simulink model "Lab3_2"  (R2016a)
settings: Solver=FixedStepDiscrete  StartTime=0.0  StopTime=10.0  RelTol=1e-3
settings Model: Creator=NoteBook  LastModifiedBy=NoteBook
settings OptimizationCC: DefaultParameterBehavior=Inlined  EnableMemcpy=off  OptimizeModelRefInitCode=on  LifeSpan=1
settings DebuggingCC: UnderspecifiedInitializationDetection=Classic  MergeDetectMultiDrivingBlocksExec=none
settings ModelReferenceCC: PropagateSignalLabelsOutOfModel=off
settings RTWCC: SystemTargetFile=ert.tlc  GenCodeOnly=on  TemplateMakefile=ert_default_tmf  GenerateReport=on  IncludeHyperlinkInReport=on  LaunchReport=on  GenerateTraceInfo=on  GenerateTraceReport=on  GenerateTraceReportSl=on  GenerateTraceReportSf=on  GenerateTraceReportEml=on
settings CodeAppCC: ForceParamTrailComments=on  IgnoreCustomStorageClasses=off  OperatorAnnotations=on  SimulinkDataObjDesc=on  SFDataObjDesc=on  MATLABFcnDesc=on  InsertBlockDesc=on  MATLABSourceComments=on
settings ERTTargetCC: GenerateSampleERTMain=on  InlinedParameterPlacement=NonHierarchical  ERTCustomFileTemplate=example_file_process.tlc

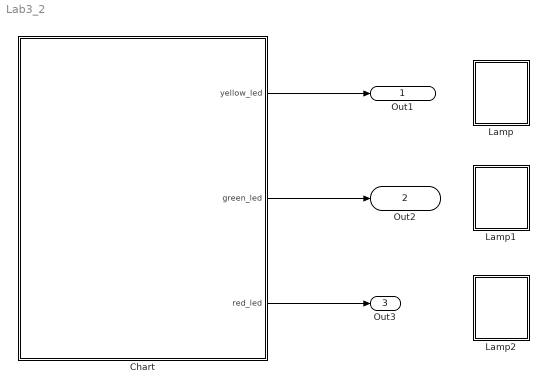
== system Lab3_2 ==
  Chart : Stateflow chart  TreatAsAtomicUnit=on
  Lamp : Subsystem  DialogController=hmiCreateDDGDialog  IsWebBlock=on  mask(MWDashboardBlock){webBlockId=2661d3e9-8543-4f99-aaf3-ccca5fb902ba, webBlockType=lamp, ShowInLibBrowser=on, ShowInitialText=on, HMISrcModelName=Lab3_2}
      mask prompts: webBlockType "WebBlock Type"; HMISrcModelName "Source Model"
      mask Help: helpview([docroot '/mapfiles/simulink.map'], 'hmi_lamp')
      mask Display:
      | if strcmp(get_param(bdroot(gcb),'BlockDiagramType'), 'library')
      |     image([(matlabroot) '/toolbox/simulink/hmi/icons/Lamp.png']);
      | end
  Lamp1 : Subsystem  DialogController=hmiCreateDDGDialog  IsWebBlock=on  mask(MWDashboardBlock){webBlockId=5fd369d1-2967-4dad-81f1-e6972ce0e81c, webBlockType=lamp, ShowInLibBrowser=on, ShowInitialText=on, HMISrcModelName=Lab3_2}
      mask prompts: webBlockType "WebBlock Type"; HMISrcModelName "Source Model"
      mask Help: helpview([docroot '/mapfiles/simulink.map'], 'hmi_lamp')
      mask Display:
      | if strcmp(get_param(bdroot(gcb),'BlockDiagramType'), 'library')
      |     image([(matlabroot) '/toolbox/simulink/hmi/icons/Lamp.png']);
      | end
  Lamp2 : Subsystem  DialogController=hmiCreateDDGDialog  IsWebBlock=on  mask(MWDashboardBlock){webBlockId=cd07f273-ba9a-41f3-9133-f6ba80ad2a34, webBlockType=lamp, ShowInLibBrowser=on, ShowInitialText=on, HMISrcModelName=Lab3_2}
      mask prompts: webBlockType "WebBlock Type"; HMISrcModelName "Source Model"
      mask Help: helpview([docroot '/mapfiles/simulink.map'], 'hmi_lamp')
      mask Display:
      | if strcmp(get_param(bdroot(gcb),'BlockDiagramType'), 'library')
      |     image([(matlabroot) '/toolbox/simulink/hmi/icons/Lamp.png']);
      | end
  Out1 : Outport  OutDataTypeStr=double
  Out2 : Outport  Port=2  OutDataTypeStr=double
  Out3 : Outport  Port=3  OutDataTypeStr=double
  wires:
  Chart/3(red_led) -> Out3/1
  Chart/2(green_led) -> Out2/1
  Chart/1(yellow_led) -> Out1/1

== system Lab3_2/Lamp ==

== system Lab3_2/Lamp1 ==

== system Lab3_2/Lamp2 ==

== stateflow chart Lab3_2/Chart ==
  state Ready
    en:
    red_led = 0;
    yellow_led = 0;
    green_led = 0;
    du:
    red_led = 0;
    yellow_led = 1;
    green_led = 0;
    ex:
  state Stop
    en:
    red_led = 0;
    yellow_led = 0;
    green_led = 0;
    du:
    red_led = 1;
    yellow_led = 0;
    green_led = 0;
    ex:
  state Go
    en:
    red_led = 0;
    yellow_led = 0;
    green_led = 0;
    du:
    red_led = 0;
    yellow_led = 0;
    green_led = 1;
    ex:
  (default) -> Ready
  Stop -> Ready : after(3000,msec)
  Go -> Stop : after(3000,msec)
  Ready -> Go : after(3000,msec)
  data: yellow_led output double size=1; green_led output double size=1; red_led output double size=1
